simulink model "punto3_simulink_parte1"  (R2024a)
settings: Solver=VariableStepAuto  StartTime=0.0  StopTime=2  RelTol=1e-3
undefined symbols (not defined in the file): A, B, C, D
settings Model: Creator=USER  LastModifiedBy=USER

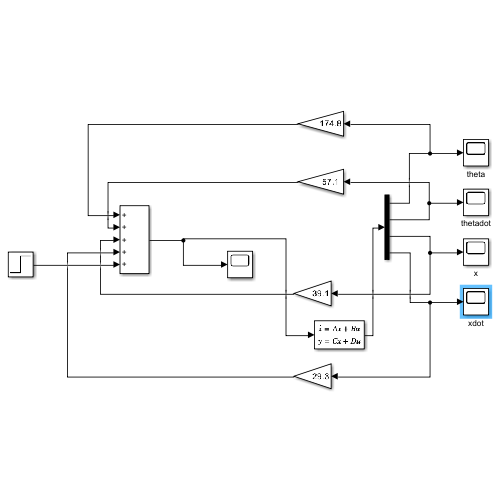
[thumbnail: Simulink's stored preview of the top-level diagram]
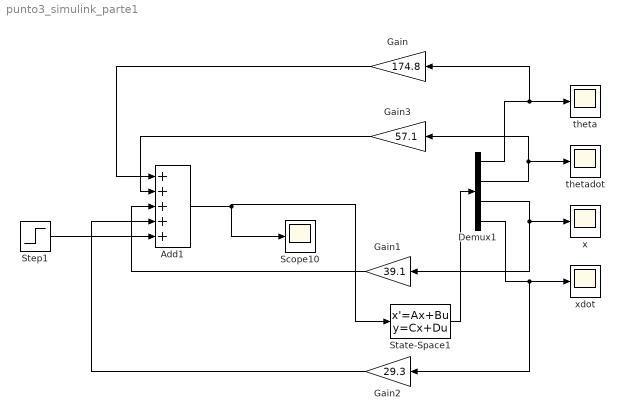
== system punto3_simulink_parte1 ==
  Add1 : Sum  Inputs=+++++
  Demux1 : Demux
  Gain : Gain  Gain=174.8
  Gain1 : Gain  Gain=39.1
  Gain2 : Gain  Gain=29.3
  Gain3 : Gain  Gain=57.1
  Scope10 : Scope
  State-Space1 : StateSpace  A=A  B=B  C=C  D=D  InitialCondition=0  ParameterTunability=Unconstrained  AllowTunableDMatrix=on
  Step1 : Step  After=10  SampleTime=0
  theta : Scope
  thetadot : Scope
  x : Scope
  xdot : Scope
  wires:
  Step1/1 -> Add1/5
  Demux1/1 -> Gain/1, theta/1
  Add1/1 -> State-Space1/1, Scope10/1
  Gain1/1 -> Add1/3
  Demux1/2 -> Gain3/1, thetadot/1
  Gain2/1 -> Add1/4
  State-Space1/1 -> Demux1/1
  Demux1/4 -> Gain2/1, xdot/1
  Gain3/1 -> Add1/2
  Demux1/3 -> Gain1/1, x/1
  Gain/1 -> Add1/1
